simulink model "sim_ca3"  (R2023b)
settings: Solver=FixedStepDiscrete  StartTime=0.0  StopTime=100  RelTol=1e-3
values from neighbouring files (symbols this model uses):
  kc_1 = 1    [ca2_params.m]    (also in iterate_gains.m)
  kI_1 = 1    [ca2_params.m]    (also in iterate_gains.m)
undefined symbols (not defined in the file or in its folder): DiscIntNeverNeededParam
settings Model: Creator=john  LastModifiedBy=john

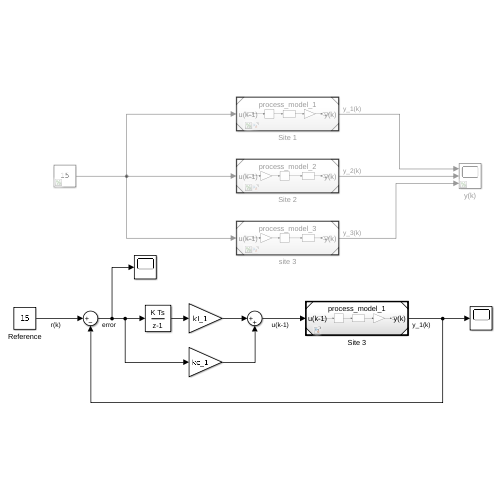
[thumbnail: Simulink's stored preview of the top-level diagram]
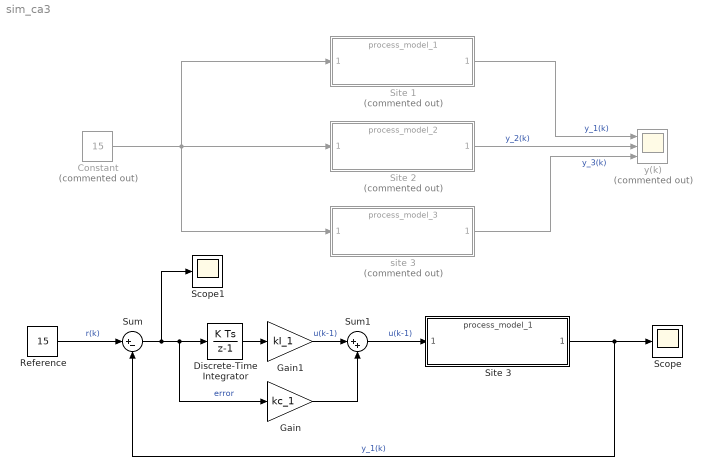
== system sim_ca3 ==
  Constant : Constant  Commented=on  Value=15
  Discrete-Time Integrator : DiscreteIntegrator  SampleTime=-1  ICPrevOutput=DiscIntNeverNeededParam  ICPrevScaledInput=DiscIntNeverNeededParam
  Gain : Gain  Gain=kc_1
  Gain1 : Gain  Gain=kI_1
  Reference : Constant  Value=15
  Scope : Scope
  Scope1 : Scope
  Site 1 : ModelReference  Commented=on  ModelNameDialog=process_model_1.slx  SimulationMode=Normal  ModelReferenceVersion=1.6
  Site 2 : ModelReference  Commented=on  ModelNameDialog=process_model_2.slx  SimulationMode=Normal  ModelReferenceVersion=1.5
  Site 3 : ModelReference  ModelNameDialog=process_model_1.slx  SimulationMode=Normal  ModelReferenceVersion=1.6
  Sum : Sum  Inputs=|+-
  Sum1 : Sum  Inputs=|++
  site 3 : ModelReference  Commented=on  ModelNameDialog=process_model_3.slx  SimulationMode=Normal  ModelReferenceVersion=1.4
  y(k) : Scope  Commented=on  NumInputPorts=3
  wires:
  Constant/1 -> Site 2/1, site 3/1, Site 1/1
  Site 1/1 -> y(k)/1  "y_1(k)"
  Site 2/1 -> y(k)/2  "y_2(k)"
  site 3/1 -> y(k)/3  "y_3(k)"
  Sum/1 -> Scope1/1, Discrete-Time Integrator/1, Gain/1  "error"
  Gain/1 -> Sum1/2
  Site 3/1 -> Scope/1, Sum/2  "y_1(k)"
  Reference/1 -> Sum/1  "r(k)"
  Discrete-Time Integrator/1 -> Gain1/1
  Gain1/1 -> Sum1/1  "u(k-1)"
  Sum1/1 -> Site 3/1  "u(k-1)"
